simulink library "SimulinkLibrary"  (R2021b)
settings: Solver=VariableStepAuto  StartTime=0.0  StopTime=10.0  RelTol=1e-3
undefined symbols (not defined in the file): Ts, w0
libraries: canmsglib x6, $bdroot x5, sharedtransform x2, simulink x1
(part 1 of 3)
settings Model: Creator=mujim  LastModifiedBy=MujtabaMusa
settings SolverCC: AlgebraicLoopSolver=TrustRegion
settings DebuggingCC: SFMachineParentedDataDiag=warning

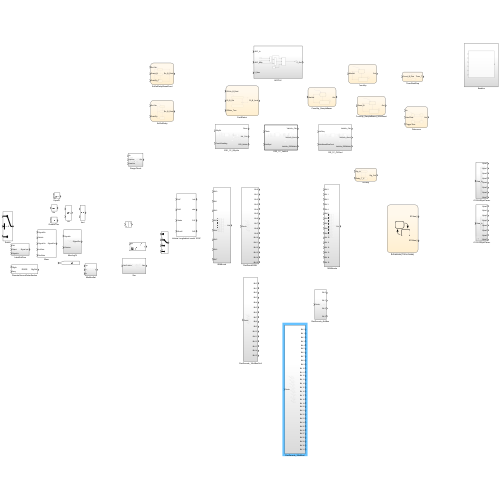
[thumbnail: Simulink's stored preview of the top-level diagram]
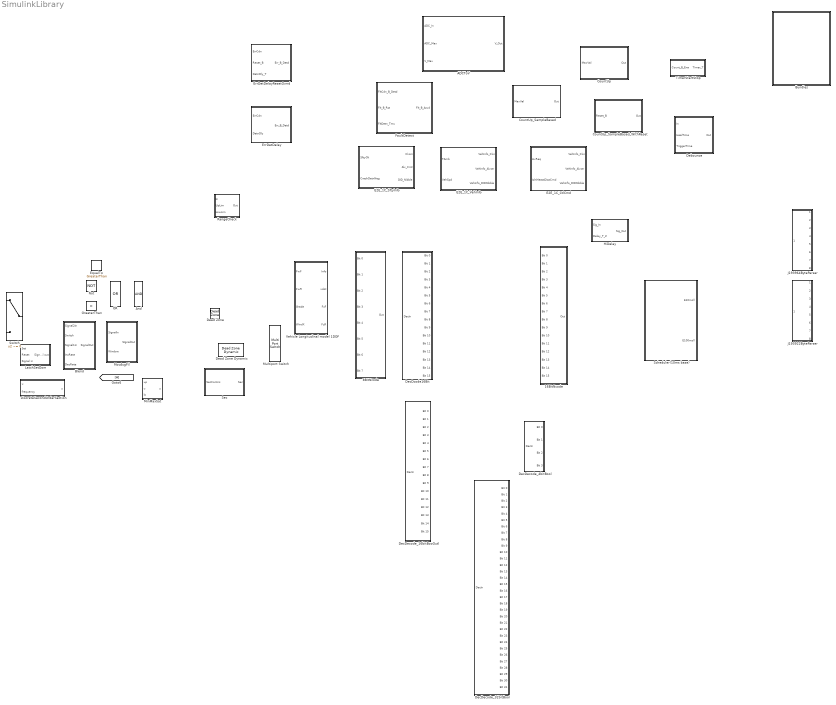
== system SimulinkLibrary ==
  16BitNcode : Subsystem
  8BitNcode : Subsystem
  ADCToV : Subsystem
  And : Logic  AllPortsSameDT=off  OutDataTypeStr=boolean
  Blend : Subsystem  Description=|
      | Blend between 2 signals with a defined rate of rise and fall
      | Switch input:
      | 0 = Signal1
      | 1 = Signal2
      | 
      | Rate is per time step
      mask help:
      | Blend between 2 signals with a defined rate of rise and fall
      | Switch input:
      | 0 = Signal1
      | 1 = Signal2
      |
      | Rate is per time step
      |
      | Use requires a stateflow license
  Bundles : Subsystem
  CountUp : Stateflow chart  TreatAsAtomicUnit=on
  CountUp_SampleBased : Stateflow chart  TreatAsAtomicUnit=on
  CountUp_SampleBased_WithReset : Stateflow chart  TreatAsAtomicUnit=on
  Dead Zone : DeadZone  SaturateOnIntegerOverflow=on
  Dead Zone Dynamic : simulink/Discontinuities/Dead Zone Dynamic
      settings: SourceProductBaseCode=SL
  Debounce : Stateflow chart  TreatAsAtomicUnit=on
  DecDcode16Bit : Subsystem
  DecDecode_16bitBooOutl : Subsystem
  DecDecode_32bitBool : Subsystem
  DecDecode_4bitBool : Subsystem
  DiscreteSecondOrderSection : Subsystem  mask(DiscreteSecondOrderSection){zeta=sin(1*pi/4), Ts=Ts, w0=w0}
      mask prompts: zeta "Damping ratio"; Ts "Sample time Ts"; w0 "Pre-warping frequency w0"
      mask help:
      | Implements the Tustin discretization of the second-order lowpass filter
      |
      |                          w^2
      | F(s) = ---------------------------------------
      |            s^2 + 2 * zeta * w * s + w^2
      |
      | where zeta is the damping ratio and w is the cutoff frequency value fed to the "frequency" port. The discrete transfer function is obtained by Tustin transformation with pre-warping at the frequency w0. The default value w0=0 corresponds to the usual bilinear transformation:
      |
      | s = 2/Ts (z-1)/(z+1).
      mask init:
      | if w0>0
      |    tau = tan(w0*Ts/2)/w0;
      | else
      |    tau = Ts/2;
      | end
      mask Display:
      | text(0.4,0.5,'DSOS');
      | port_label('input', 1, 'SigIn');
      | port_label('output', 1, 'SigOut');
      | port_label('input', 2, 'freq');
  E2E_1C_CtlCmd : Subsystem
  E2E_1C_SftyInfo : Subsystem
  E2E_1C_VehInfo : Subsystem  TreatAsAtomicUnit=on
  EqualTo : $bdroot/GreaterThan  Operator===  OutDataTypeStr=boolean  SampleTime=-1  RndMeth=Zero
  ErrDetDelay : Stateflow chart  TreatAsAtomicUnit=on
  ErrDetDelayResetOvrrd : Stateflow chart  TreatAsAtomicUnit=on
  FaultDetect : Stateflow chart  TreatAsAtomicUnit=on
  GreaterThan : RelationalOperator  Operator=>  OutDataTypeStr=boolean  RndMeth=Zero
  HiDelay : Stateflow chart  TreatAsAtomicUnit=on
  J193922ByteParser : Subsystem  AncestorBlock=SimulinkLibrary/J193964ByteParser
  J193964ByteParser : Subsystem
  LatchSetDom : Subsystem
  MinMaxSat : Subsystem
  MovAvgFil : Subsystem
  Multiport Switch : MultiPortSwitch  Inputs=2  DataPortForDefault=Additional data port  DiagnosticForDefault=None  RndMeth=Zero
  Not : Logic  Operator=NOT  OutDataTypeStr=boolean
  OR : Logic  Operator=OR  AllPortsSameDT=off  OutDataTypeStr=boolean
  RangeCheck : Subsystem
  Scheduler(10ms base) : Stateflow chart  TreatAsAtomicUnit=on
      settings: RTWMemSecFuncInitTerm=Default  RTWMemSecFuncExecute=Default
  Sec : Subsystem
  Switch : Switch  Criteria=u2 ~= 0  OutDataTypeStr=double  RndMeth=Zero
  TimerStartStop : Stateflow chart  TreatAsAtomicUnit=on
  Vehicle Longitudinal model 1DOF : Subsystem  mask(Vehicle Longitudinal model 1DOF){NF=0, NR=0, m=0, a=0, b=0, h=0, Cd=0, Cl=0, Cpm=0, Af=0, x_o=0, xdot_o=0, Pabs=0, T=0, g=0}
      mask prompts: NF "Number of wheels on front axle, NF [-]"; NR "Number of wheels on rear axle, NR [-]"; m "Mass, m [Kg]"; a "Horizontal distance from CG to front axle, a [m]"; b "Horizontal distance from CG to rear axle, b [m]"; h "CG height above axles, h [m]"; Cd "Drag coefficient, Cd [-]"; Cl "Lift coefficient, Cl [-]"; Cpm "Pitch drag moment coeffiecient, Cpm [-]"; Af "Frontal Area, Af [m^2]"; x_o "Initial position, x_o [m]"; xdot_o "Initial velocity, xdot_o [m/s]"; Pabs "Absolute Pressure, Pabs [Pa]"; T "Air Temp, T [K]"; g "Gravitational acceleration, g [m/s^2]"
      mask DialogControl Container3 Prompt: Parameters
      mask DialogControl Container4 Prompt: Vehicle Paramters
      mask DialogControl Container11 Prompt: Environmental Parameters

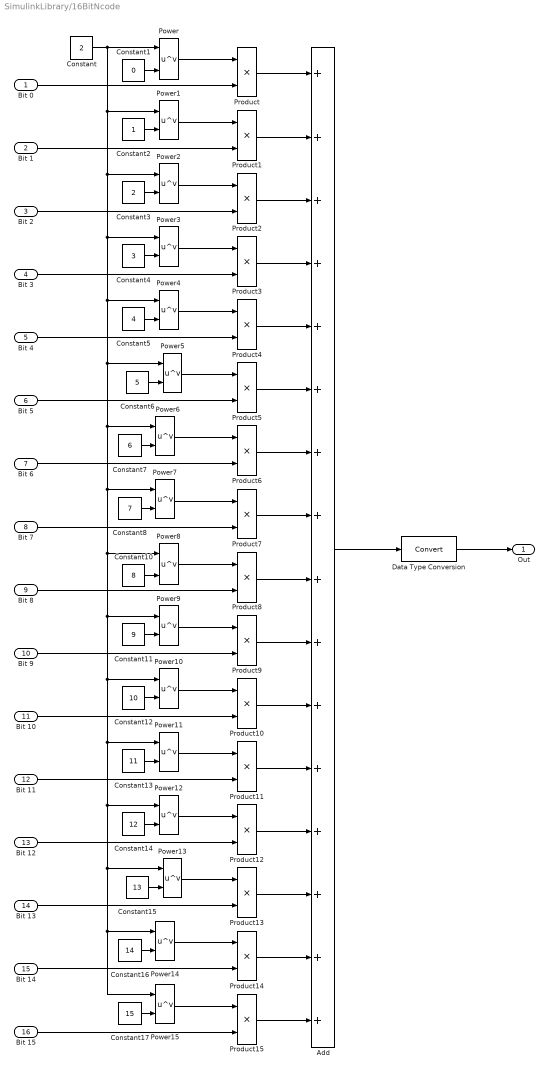
== system SimulinkLibrary/16BitNcode ==
  Bit 0 : Inport  OutDataTypeStr=boolean
  Bit 1 : Inport  Port=2  OutDataTypeStr=boolean
  Bit 2 : Inport  Port=3  OutDataTypeStr=boolean
  Bit 3 : Inport  Port=4  OutDataTypeStr=boolean
  Bit 4 : Inport  Port=5  OutDataTypeStr=boolean
  Bit 5 : Inport  Port=6  OutDataTypeStr=boolean
  Bit 6 : Inport  Port=7  OutDataTypeStr=boolean
  Bit 7 : Inport  Port=8  OutDataTypeStr=boolean
  Bit 8 : Inport  Port=9  OutDataTypeStr=boolean
  Bit 9 : Inport  Port=10  OutDataTypeStr=boolean
  Bit 10 : Inport  Port=11  OutDataTypeStr=boolean
  Bit 11 : Inport  Port=12  OutDataTypeStr=boolean
  Bit 12 : Inport  Port=13  OutDataTypeStr=boolean
  Bit 13 : Inport  Port=14  OutDataTypeStr=boolean
  Bit 14 : Inport  Port=15  OutDataTypeStr=boolean
  Bit 15 : Inport  Port=16  OutDataTypeStr=boolean
  Add : Sum  Inputs=++++++++++++++++
  Constant : Constant  Value=2  OutDataTypeStr=single
  Constant1 : Constant  Value=0  OutDataTypeStr=single
  Constant10 : Constant  Value=8  OutDataTypeStr=single
  Constant11 : Constant  Value=9  OutDataTypeStr=single
  Constant12 : Constant  Value=10  OutDataTypeStr=single
  Constant13 : Constant  Value=11  OutDataTypeStr=single
  Constant14 : Constant  Value=12  OutDataTypeStr=single
  Constant15 : Constant  Value=13  OutDataTypeStr=single
  Constant16 : Constant  Value=14  OutDataTypeStr=single
  Constant17 : Constant  Value=15  OutDataTypeStr=single
  Constant2 : Constant  OutDataTypeStr=single
  Constant3 : Constant  Value=2  OutDataTypeStr=single
  Constant4 : Constant  Value=3  OutDataTypeStr=single
  Constant5 : Constant  Value=4  OutDataTypeStr=single
  Constant6 : Constant  Value=5  OutDataTypeStr=single
  Constant7 : Constant  Value=6  OutDataTypeStr=single
  Constant8 : Constant  Value=7  OutDataTypeStr=single
  Data Type Conversion : DataTypeConversion
  Power{,1..15} (16 alike) : Math  Operator=pow  SaturateOnIntegerOverflow=on
  Product{,1..15} (16 alike) : Product
  Out : Outport
  wires:
  Bit 6/1 -> Product6/2
  Bit 5/1 -> Product5/2
  Product1/1 -> Add/2
  Product/1 -> Add/1
  Bit 1/1 -> Product1/2
  Product7/1 -> Add/8
  Power2/1 -> Product2/1
  Power7/1 -> Product7/1
  Power4/1 -> Product4/1
  Power1/1 -> Product1/1
  Power3/1 -> Product3/1
  Constant4/1 -> Power3/2
  Constant2/1 -> Power1/2
  Constant6/1 -> Power5/2
  Bit 7/1 -> Product7/2
  Constant3/1 -> Power2/2
  Bit 3/1 -> Product3/2
  Bit 4/1 -> Product4/2
  Add/1 -> Data Type Conversion/1
  Power6/1 -> Product6/1
  Constant1/1 -> Power/2
  Bit 2/1 -> Product2/2
  Power5/1 -> Product5/1
  Constant8/1 -> Power7/2
  Bit 0/1 -> Product/2
  Product3/1 -> Add/4
  Product2/1 -> Add/3
  Product4/1 -> Add/5
  Product6/1 -> Add/7
  Constant7/1 -> Power6/2
  Data Type Conversion/1 -> Out/1
  Product5/1 -> Add/6
  Power/1 -> Product/1
  Constant5/1 -> Power4/2
  Product12/1 -> Add/13
  Constant16/1 -> Power14/2
  Product13/1 -> Add/14
  Power8/1 -> Product8/1
  Constant17/1 -> Power15/2
  Product10/1 -> Add/11
  Product11/1 -> Add/12
  Constant14/1 -> Power12/2
  Power13/1 -> Product13/1
  Constant15/1 -> Power13/2
  Constant12/1 -> Power10/2
  Constant/1 -> Power/1, Power1/1, Power2/1, Power3/1, Power8/1, Power9/1, Power10/1, Power11/1, Power15/1, Power14/1, Power13/1, Power12/1, Power7/1, Power6/1, Power5/1, Power4/1
  Product14/1 -> Add/15
  Constant13/1 -> Power11/2
  Constant11/1 -> Power9/2
  Bit 10/1 -> Product10/2
  Power11/1 -> Product11/1
  Constant10/1 -> Power8/2
  Power12/1 -> Product12/1
  Power9/1 -> Product9/1
  Bit 12/1 -> Product12/2
  Power15/1 -> Product15/1
  Bit 15/1 -> Product15/2
  Bit 11/1 -> Product11/2
  Power10/1 -> Product10/1
  Bit 9/1 -> Product9/2
  Product15/1 -> Add/16
  Product9/1 -> Add/10
  Power14/1 -> Product14/1
  Bit 13/1 -> Product13/2
  Bit 14/1 -> Product14/2
  Product8/1 -> Add/9
  Bit 8/1 -> Product8/2

== system SimulinkLibrary/8BitNcode ==
  Bit 0 : Inport  OutDataTypeStr=boolean
  Bit 1 : Inport  Port=2  OutDataTypeStr=boolean
  Bit 2 : Inport  Port=3  OutDataTypeStr=boolean
  Bit 3 : Inport  Port=4  OutDataTypeStr=boolean
  Bit 4 : Inport  Port=5  OutDataTypeStr=boolean
  Bit 5 : Inport  Port=6  OutDataTypeStr=boolean
  Bit 6 : Inport  Port=7  OutDataTypeStr=boolean
  Bit 7 : Inport  Port=8  OutDataTypeStr=boolean
  Add : Sum  Inputs=++++++++
  Constant : Constant  Value=2  OutDataTypeStr=single
  Constant1 : Constant  Value=0  OutDataTypeStr=single
  Constant2 : Constant  OutDataTypeStr=single
  Constant3 : Constant  Value=2  OutDataTypeStr=single
  Constant4 : Constant  Value=3  OutDataTypeStr=single
  Constant5 : Constant  Value=4  OutDataTypeStr=single
  Constant6 : Constant  Value=5  OutDataTypeStr=single
  Constant7 : Constant  Value=6  OutDataTypeStr=single
  Constant8 : Constant  Value=7  OutDataTypeStr=single
  Data Type Conversion : DataTypeConversion
  Power{,1..7} (8 alike) : Math  Operator=pow  SaturateOnIntegerOverflow=on
  Product{,1..7} (8 alike) : Product
  Out : Outport
  wires:
  Bit 0/1 -> Product/2
  Constant/1 -> Power/1, Power1/1, Power2/1, Power3/1, Power7/1, Power6/1, Power5/1, Power4/1
  Power/1 -> Product/1
  Add/1 -> Data Type Conversion/1
  Constant1/1 -> Power/2
  Constant2/1 -> Power1/2
  Constant3/1 -> Power2/2
  Constant4/1 -> Power3/2
  Constant5/1 -> Power4/2
  Constant6/1 -> Power5/2
  Constant7/1 -> Power6/2
  Constant8/1 -> Power7/2
  Product/1 -> Add/1
  Product1/1 -> Add/2
  Product2/1 -> Add/3
  Product3/1 -> Add/4
  Product4/1 -> Add/5
  Product5/1 -> Add/6
  Product6/1 -> Add/7
  Product7/1 -> Add/8
  Power1/1 -> Product1/1
  Power2/1 -> Product2/1
  Power3/1 -> Product3/1
  Power4/1 -> Product4/1
  Power5/1 -> Product5/1
  Power6/1 -> Product6/1
  Power7/1 -> Product7/1
  Bit 1/1 -> Product1/2
  Bit 2/1 -> Product2/2
  Bit 3/1 -> Product3/2
  Bit 4/1 -> Product4/2
  Bit 5/1 -> Product5/2
  Bit 6/1 -> Product6/2
  Bit 7/1 -> Product7/2
  Data Type Conversion/1 -> Out/1

== system SimulinkLibrary/ADCToV ==
  ADC_In : Inport
  ADC_Max : Inport  Port=2
  V_Max : Inport  Port=3
  Constant : Constant  Value=0
  Divide : Product  Inputs=*/
  MinMaxSat : $bdroot/MinMaxSat  SystemSampleTime=-1  VariantActivationTime=update diagram  Latency=0  AutoFrameSizeCalculation=off
  Product : Product
  V_Out : Outport
  wires:
  Constant/1 -> MinMaxSat/3
  MinMaxSat/1 -> V_Out/1  "V_Out"
  Product/1 -> MinMaxSat/2
  V_Max/1 -> Product/2, MinMaxSat/1  "V_Max"
  Divide/1 -> Product/1
  ADC_In/1 -> Divide/1  "ADC_In"
  ADC_Max/1 -> Divide/2  "ADC_Max"

== system SimulinkLibrary/Blend ==
  note: Blend between 2 signals with a defined rate of rise and fall
      | Switch input:
      | 0 = Signal1
      | 1 = Signal2
      |
      | Rate is per time step
  Signal2In : Inport
  Switch : Inport  Port=2
  Signal1In : Inport  Port=3
  IncRate : Inport  Port=4
  DecRate : Inport  Port=5
  Chart : Stateflow chart  TreatAsAtomicUnit=on
  SignalOut : Outport
  wires:
  Signal2In/1 -> Chart/3(SigIn2)
  Signal1In/1 -> Chart/2(SigIn1)
  DecRate/1 -> Chart/5(DecRate)
  Switch/1 -> Chart/1(Swt)
  IncRate/1 -> Chart/4(IncRate)
  Chart/1(SigOut) -> SignalOut/1

== system SimulinkLibrary/Bundles ==
  HwSelProc : Subsystem

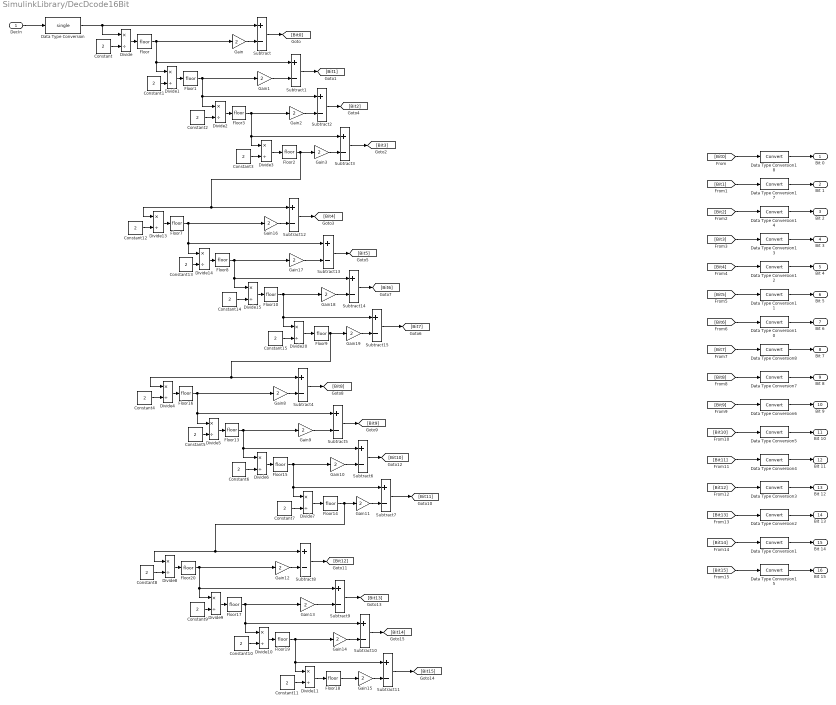
== system SimulinkLibrary/DecDcode16Bit ==
  DecIn : Inport
  Constant{,1..15} (16 alike) : Constant  Value=2  OutDataTypeStr=single
  Data Type Conversion : DataTypeConversion  OutDataTypeStr=single
  Data Type Conversion{1..8,10..15,17..18} (16 alike) : DataTypeConversion
  Divide{,1..11,13..15,20} (16 alike) : Product  Inputs=*/  OutDataTypeStr=Inherit: Inherit via back propagation
  Floor{,1..3,7..10,13..20} (16 alike) : Rounding
  Gain{,1..3,8..19} (16 alike) : Gain  Gain=2
  Subtract{,1..15} (16 alike) : Sum  Inputs=+-
  Bit 0 : Outport
  Bit 1 : Outport  Port=2
  Bit 2 : Outport  Port=3
  Bit 3 : Outport  Port=4
  Bit 4 : Outport  Port=5
  Bit 5 : Outport  Port=6
  Bit 6 : Outport  Port=7
  Bit 7 : Outport  Port=8
  Bit 8 : Outport  Port=9
  Bit 9 : Outport  Port=10
  Bit 10 : Outport  Port=11
  Bit 11 : Outport  Port=12
  Bit 12 : Outport  Port=13
  Bit 13 : Outport  Port=14
  Bit 14 : Outport  Port=15
  Bit 15 : Outport  Port=16
  wires:
  Constant/1 -> Divide/2
  Divide/1 -> Floor/1
  Divide1/1 -> Floor1/1
  Constant1/1 -> Divide1/2
  Subtract/1 -> [Bit0]
  Constant2/1 -> Divide2/2
  Divide2/1 -> Floor3/1
  [Bit0] -> Data Type Conversion18/1
  Subtract1/1 -> [Bit1]
  [Bit1] -> Data Type Conversion17/1
  Subtract3/1 -> [Bit3]
  Constant3/1 -> Divide3/2
  Subtract2/1 -> [Bit2]
  [Bit2] -> Data Type Conversion14/1
  [Bit3] -> Data Type Conversion13/1
  [Bit4] -> Data Type Conversion12/1
  [Bit5] -> Data Type Conversion11/1
  [Bit6] -> Data Type Conversion10/1
  [Bit7] -> Data Type Conversion8/1
  [Bit15] -> Data Type Conversion15/1
  [Bit14] -> Data Type Conversion1/1
  [Bit13] -> Data Type Conversion2/1
  [Bit12] -> Data Type Conversion3/1
  [Bit11] -> Data Type Conversion4/1
  [Bit10] -> Data Type Conversion5/1
  [Bit9] -> Data Type Conversion6/1
  [Bit8] -> Data Type Conversion7/1
  Gain/1 -> Subtract/2
  Gain1/1 -> Subtract1/2
  Gain2/1 -> Subtract2/2
  Gain3/1 -> Subtract3/2
  Divide3/1 -> Floor2/1
  Data Type Conversion18/1 -> Bit 0/1
  Data Type Conversion17/1 -> Bit 1/1
  Data Type Conversion14/1 -> Bit 2/1
  Data Type Conversion13/1 -> Bit 3/1
  Data Type Conversion12/1 -> Bit 4/1
  Data Type Conversion11/1 -> Bit 5/1
  Data Type Conversion10/1 -> Bit 6/1
  Data Type Conversion8/1 -> Bit 7/1
  Data Type Conversion7/1 -> Bit 8/1
  Data Type Conversion6/1 -> Bit 9/1
  Data Type Conversion5/1 -> Bit 10/1
  Data Type Conversion4/1 -> Bit 11/1
  Data Type Conversion3/1 -> Bit 12/1
  Data Type Conversion2/1 -> Bit 13/1
  Data Type Conversion1/1 -> Bit 14/1
  Data Type Conversion15/1 -> Bit 15/1
  DecIn/1 -> Data Type Conversion/1
  Floor/1 -> Gain/1, Divide1/1, Subtract1/1
  Floor1/1 -> Gain1/1, Divide2/1, Subtract2/1
  Floor3/1 -> Gain2/1, Divide3/1, Subtract3/1
  Floor10/1 -> Subtract15/1, Divide20/1, Gain18/1
  Floor8/1 -> Subtract14/1, Divide15/1, Gain17/1
  Floor7/1 -> Subtract13/1, Divide14/1, Gain16/1
  Floor2/1 -> Divide13/1, Subtract12/1, Gain3/1
  Divide20/1 -> Floor9/1
  Gain19/1 -> Subtract15/2
  Gain18/1 -> Subtract14/2
  Gain17/1 -> Subtract13/2
  Gain16/1 -> Subtract12/2
  Subtract14/1 -> [Bit6]
  Constant15/1 -> Divide20/2
  Subtract15/1 -> [Bit7]
  Subtract13/1 -> [Bit5]
  Divide15/1 -> Floor10/1
  Constant14/1 -> Divide15/2
  Subtract12/1 -> [Bit4]
  Constant13/1 -> Divide14/2
  Divide14/1 -> Floor8/1
  Divide13/1 -> Floor7/1
  Constant12/1 -> Divide13/2
  Floor15/1 -> Subtract7/1, Divide7/1, Gain10/1
  Floor13/1 -> Subtract6/1, Divide6/1, Gain9/1
  Floor16/1 -> Subtract5/1, Divide5/1, Gain8/1
  Floor9/1 -> Gain19/1, Divide4/1, Subtract4/1
  Divide7/1 -> Floor14/1
  Gain11/1 -> Subtract7/2
  Gain10/1 -> Subtract6/2
  Gain9/1 -> Subtract5/2
  Gain8/1 -> Subtract4/2
  Subtract6/1 -> [Bit10]
  Constant7/1 -> Divide7/2
  Subtract7/1 -> [Bit11]
  Subtract5/1 -> [Bit9]
  Divide6/1 -> Floor15/1
  Constant6/1 -> Divide6/2
  Subtract4/1 -> [Bit8]
  Constant5/1 -> Divide5/2
  Divide5/1 -> Floor13/1
  Divide4/1 -> Floor16/1
  Constant4/1 -> Divide4/2
  Floor18/1 -> Gain15/1
  Floor19/1 -> Subtract11/1, Divide11/1, Gain14/1
  Floor17/1 -> Subtract10/1, Divide10/1, Gain13/1
  Floor20/1 -> Subtract9/1, Divide9/1, Gain12/1
  Floor14/1 -> Subtract8/1, Divide8/1, Gain11/1
  Divide11/1 -> Floor18/1
  Gain15/1 -> Subtract11/2
  Gain14/1 -> Subtract10/2
  Gain13/1 -> Subtract9/2
  Gain12/1 -> Subtract8/2
  Subtract10/1 -> [Bit14]
  Constant11/1 -> Divide11/2
  Subtract11/1 -> [Bit15]
  Subtract9/1 -> [Bit13]
  Divide10/1 -> Floor19/1
  Constant10/1 -> Divide10/2
  Subtract8/1 -> [Bit12]
  Constant9/1 -> Divide9/2
  Divide9/1 -> Floor17/1
  Divide8/1 -> Floor20/1
  Constant8/1 -> Divide8/2
  Data Type Conversion/1 -> Divide/1, Subtract/1

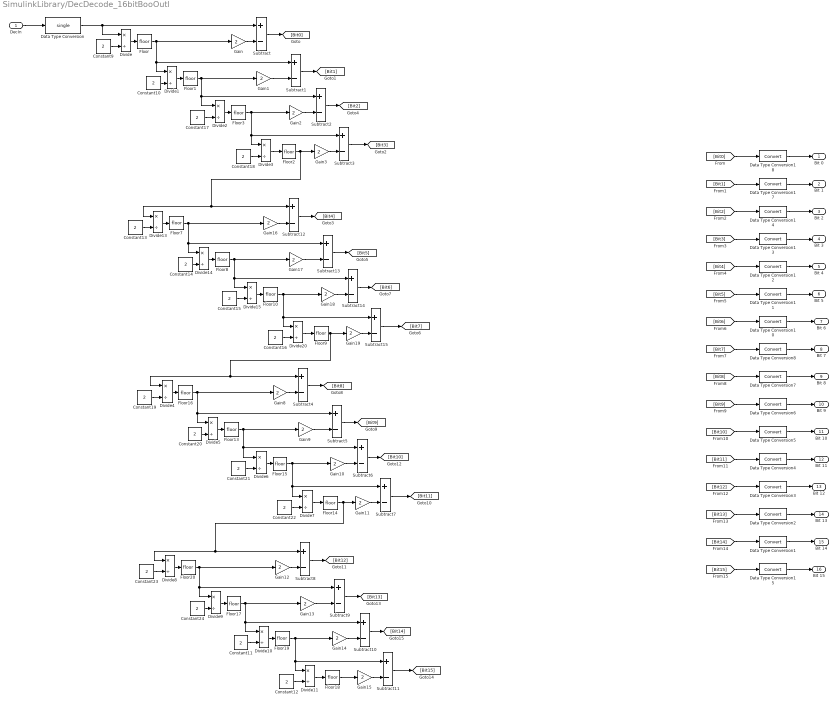
== system SimulinkLibrary/DecDecode_16bitBooOutl ==
  DecIn : Inport
  Constant{9..24} (16 alike) : Constant  Value=2  OutDataTypeStr=single
  Data Type Conversion : DataTypeConversion  OutDataTypeStr=single
  Data Type Conversion{1..8,10..15,17..18} (16 alike) : DataTypeConversion
  Divide{,1..11,13..15,20} (16 alike) : Product  Inputs=*/  OutDataTypeStr=Inherit: Inherit via back propagation
  Floor{,1..3,7..10,13..20} (16 alike) : Rounding
  Gain{,1..3,8..19} (16 alike) : Gain  Gain=2
  Subtract{,1..15} (16 alike) : Sum  Inputs=+-
  Bit 0 : Outport  OutDataTypeStr=boolean
  Bit 1 : Outport  Port=2  OutDataTypeStr=boolean
  Bit 2 : Outport  Port=3  OutDataTypeStr=boolean
  Bit 3 : Outport  Port=4  OutDataTypeStr=boolean
  Bit 4 : Outport  Port=5  OutDataTypeStr=boolean
  Bit 5 : Outport  Port=6  OutDataTypeStr=boolean
  Bit 6 : Outport  Port=7  OutDataTypeStr=boolean
  Bit 7 : Outport  Port=8  OutDataTypeStr=boolean
  Bit 8 : Outport  Port=9  OutDataTypeStr=boolean
  Bit 9 : Outport  Port=10  OutDataTypeStr=boolean
  Bit 10 : Outport  Port=11  OutDataTypeStr=boolean
  Bit 11 : Outport  Port=12  OutDataTypeStr=boolean
  Bit 12 : Outport  Port=13  OutDataTypeStr=boolean
  Bit 13 : Outport  Port=14  OutDataTypeStr=boolean
  Bit 14 : Outport  Port=15  OutDataTypeStr=boolean
  Bit 15 : Outport  Port=16  OutDataTypeStr=boolean
  wires:
  Subtract15/1 -> [Bit7]
  Gain19/1 -> Subtract15/2
  Data Type Conversion17/1 -> Bit 1/1
  Floor8/1 -> Gain17/1, Divide15/1, Subtract14/1
  Gain/1 -> Subtract/2
  Gain17/1 -> Subtract13/2
  Data Type Conversion12/1 -> Bit 4/1
  Subtract9/1 -> [Bit13]
  Divide9/1 -> Floor17/1
  Subtract1/1 -> [Bit1]
  [Bit11] -> Data Type Conversion4/1
  [Bit5] -> Data Type Conversion11/1
  [Bit9] -> Data Type Conversion6/1
  Gain1/1 -> Subtract1/2
  Subtract2/1 -> [Bit2]
  [Bit14] -> Data Type Conversion1/1
  [Bit0] -> Data Type Conversion18/1
  Data Type Conversion14/1 -> Bit 2/1
  Subtract8/1 -> [Bit12]
  Subtract7/1 -> [Bit11]
  [Bit2] -> Data Type Conversion14/1
  [Bit15] -> Data Type Conversion15/1
  Constant10/1 -> Divide1/2
  Subtract/1 -> [Bit0]
  Constant18/1 -> Divide3/2
  Constant16/1 -> Divide20/2
  [Bit1] -> Data Type Conversion17/1
  [Bit10] -> Data Type Conversion5/1
  Divide/1 -> Floor/1
  [Bit3] -> Data Type Conversion13/1
  Constant17/1 -> Divide2/2
  Floor2/1 -> Gain3/1, Subtract12/1, Divide13/1
  Data Type Conversion3/1 -> Bit 12/1
  Data Type Conversion15/1 -> Bit 15/1
  Subtract6/1 -> [Bit10]
  Constant14/1 -> Divide14/2
  Constant15/1 -> Divide15/2
  Gain13/1 -> Subtract9/2
  DecIn/1 -> Data Type Conversion/1
  Subtract5/1 -> [Bit9]
  Floor1/1 -> Subtract2/1, Divide2/1, Gain1/1
  Divide10/1 -> Floor19/1
  Divide13/1 -> Floor7/1
  Data Type Conversion2/1 -> Bit 13/1
  Gain15/1 -> Subtract11/2
  Floor13/1 -> Gain9/1, Divide6/1, Subtract6/1
  Subtract11/1 -> [Bit15]
  Constant19/1 -> Divide4/2
  Constant12/1 -> Divide11/2
  Divide5/1 -> Floor13/1
  Data Type Conversion8/1 -> Bit 7/1
  Floor18/1 -> Gain15/1
  Divide20/1 -> Floor9/1
  Constant20/1 -> Divide5/2
  Floor7/1 -> Gain16/1, Divide14/1, Subtract13/1
  Gain18/1 -> Subtract14/2
  Data Type Conversion1/1 -> Bit 14/1
  Data Type Conversion13/1 -> Bit 3/1
  Divide11/1 -> Floor18/1
  Divide7/1 -> Floor14/1
  Data Type Conversion5/1 -> Bit 10/1
  Data Type Conversion4/1 -> Bit 11/1
  Subtract13/1 -> [Bit5]
  Data Type Conversion7/1 -> Bit 8/1
  Gain3/1 -> Subtract3/2
  Constant22/1 -> Divide7/2
  Data Type Conversion11/1 -> Bit 5/1
  [Bit7] -> Data Type Conversion8/1
  Divide1/1 -> Floor1/1
  Data Type Conversion18/1 -> Bit 0/1
  Divide3/1 -> Floor2/1
  Data Type Conversion10/1 -> Bit 6/1
  Floor/1 -> Subtract1/1, Divide1/1, Gain/1
  Constant9/1 -> Divide/2
  [Bit6] -> Data Type Conversion10/1
  [Bit12] -> Data Type Conversion3/1
  Gain2/1 -> Subtract2/2
  Floor15/1 -> Gain10/1, Divide7/1, Subtract7/1
  Floor9/1 -> Subtract4/1, Divide4/1, Gain19/1
  Gain8/1 -> Subtract4/2
  Gain9/1 -> Subtract5/2
  Gain10/1 -> Subtract6/2
  Floor16/1 -> Gain8/1, Divide5/1, Subtract5/1
  Gain16/1 -> Subtract12/2
  Divide15/1 -> Floor10/1
  Floor10/1 -> Gain18/1, Divide20/1, Subtract15/1
  Floor14/1 -> Gain11/1, Divide8/1, Subtract8/1
  Subtract10/1 -> [Bit14]
  Divide14/1 -> Floor8/1
  Floor20/1 -> Gain12/1, Divide9/1, Subtract9/1
  Floor3/1 -> Subtract3/1, Divide3/1, Gain2/1
  Constant24/1 -> Divide9/2
  Divide2/1 -> Floor3/1
  Divide6/1 -> Floor15/1
  Floor17/1 -> Gain13/1, Divide10/1, Subtract10/1
  Constant13/1 -> Divide13/2
  [Bit8] -> Data Type Conversion7/1
  Gain14/1 -> Subtract10/2
  [Bit4] -> Data Type Conversion12/1
  Constant11/1 -> Divide10/2
  Subtract4/1 -> [Bit8]
  Floor19/1 -> Gain14/1, Divide11/1, Subtract11/1
  Constant21/1 -> Divide6/2
  Subtract12/1 -> [Bit4]
  Subtract3/1 -> [Bit3]
  Divide4/1 -> Floor16/1
  Data Type Conversion/1 -> Subtract/1, Divide/1
  [Bit13] -> Data Type Conversion2/1
  Divide8/1 -> Floor20/1
  Gain12/1 -> Subtract8/2
  Data Type Conversion6/1 -> Bit 9/1
  Gain11/1 -> Subtract7/2
  Subtract14/1 -> [Bit6]
  Constant23/1 -> Divide8/2

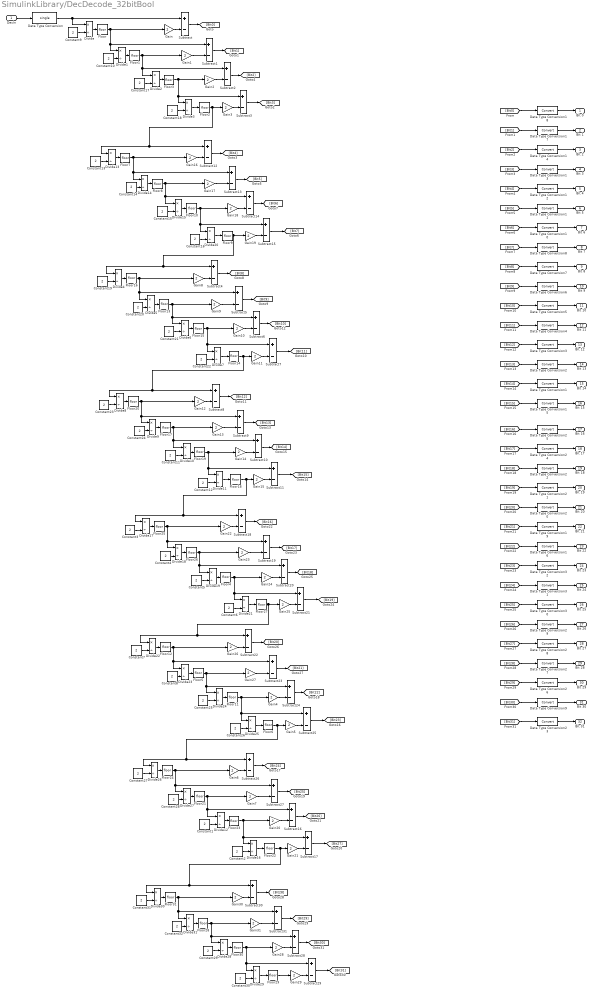
== system SimulinkLibrary/DecDecode_32bitBool ==
  DecIn : Inport
  Constant{1..32} (32 alike) : Constant  Value=2  OutDataTypeStr=single
  Data Type Conversion : DataTypeConversion  OutDataTypeStr=single
  Data Type Conversion{1..32} (32 alike) : DataTypeConversion
  Divide{,1..31} (32 alike) : Product  Inputs=*/  OutDataTypeStr=Inherit: Inherit via back propagation
  Floor{,1..31} (32 alike) : Rounding
  Gain{,1..31} (32 alike) : Gain  Gain=2
  Subtract{,1..31} (32 alike) : Sum  Inputs=+-
  Bit 0 : Outport  OutDataTypeStr=boolean
  Bit 1 : Outport  Port=2  OutDataTypeStr=boolean
  Bit 2 : Outport  Port=3  OutDataTypeStr=boolean
  Bit 3 : Outport  Port=4  OutDataTypeStr=boolean
  Bit 4 : Outport  Port=5  OutDataTypeStr=boolean
  Bit 5 : Outport  Port=6  OutDataTypeStr=boolean
  Bit 6 : Outport  Port=7  OutDataTypeStr=boolean
  Bit 7 : Outport  Port=8  OutDataTypeStr=boolean
  Bit 8 : Outport  Port=9  OutDataTypeStr=boolean
  Bit 9 : Outport  Port=10  OutDataTypeStr=boolean
  Bit 10 : Outport  Port=11  OutDataTypeStr=boolean
  Bit 11 : Outport  Port=12  OutDataTypeStr=boolean
  Bit 12 : Outport  Port=13  OutDataTypeStr=boolean
  Bit 13 : Outport  Port=14  OutDataTypeStr=boolean
  Bit 14 : Outport  Port=15  OutDataTypeStr=boolean
  Bit 15 : Outport  Port=16  OutDataTypeStr=boolean
  Bit 16 : Outport  Port=17  OutDataTypeStr=boolean
  Bit 17 : Outport  Port=18  OutDataTypeStr=boolean
  Bit 18 : Outport  Port=19  OutDataTypeStr=boolean
  Bit 19 : Outport  Port=20  OutDataTypeStr=boolean
  Bit 20 : Outport  Port=21  OutDataTypeStr=boolean
  Bit 21 : Outport  Port=22  OutDataTypeStr=boolean
  Bit 22 : Outport  Port=23  OutDataTypeStr=boolean
  Bit 23 : Outport  Port=24  OutDataTypeStr=boolean
  Bit 24 : Outport  Port=25  OutDataTypeStr=boolean
  Bit 25 : Outport  Port=26  OutDataTypeStr=boolean
  Bit 26 : Outport  Port=27  OutDataTypeStr=boolean
  Bit 27 : Outport  Port=28  OutDataTypeStr=boolean
  Bit 28 : Outport  Port=29  OutDataTypeStr=boolean
  Bit 29 : Outport  Port=30  OutDataTypeStr=boolean
  Bit 30 : Outport  Port=31  OutDataTypeStr=boolean
  Bit 31 : Outport  Port=32  OutDataTypeStr=boolean
  wires:
  Subtract4/1 -> [Bit8]
  Data Type Conversion6/1 -> Bit 9/1
  Constant23/1 -> Divide8/2
  Constant17/1 -> Divide2/2
  Constant19/1 -> Divide4/2
  Data Type Conversion13/1 -> Bit 3/1
  Floor7/1 -> Gain16/1, Divide14/1, Subtract13/1
  Divide11/1 -> Floor18/1
  Gain18/1 -> Subtract14/2
  Data Type Conversion4/1 -> Bit 11/1
  [Bit7] -> Data Type Conversion8/1
  Constant22/1 -> Divide7/2
  Constant20/1 -> Divide5/2
  Subtract11/1 -> [Bit15]
  Constant12/1 -> Divide11/2
  Data Type Conversion2/1 -> Bit 13/1
  Divide5/1 -> Floor13/1
  Gain15/1 -> Subtract11/2
  Divide10/1 -> Floor19/1
  Subtract5/1 -> [Bit9]
  Data Type Conversion15/1 -> Bit 15/1
  Gain13/1 -> Subtract9/2
  Gain17/1 -> Subtract13/2
  DecIn/1 -> Data Type Conversion/1
  [Bit10] -> Data Type Conversion5/1
  [Bit2] -> Data Type Conversion14/1
  Constant18/1 -> Divide3/2
  Subtract/1 -> [Bit0]
  Constant10/1 -> Divide1/2
  Divide/1 -> Floor/1
  Floor8/1 -> Gain17/1, Divide15/1, Subtract14/1
  [Bit1] -> Data Type Conversion17/1
  Data Type Conversion3/1 -> Bit 12/1
  [Bit11] -> Data Type Conversion4/1
  Subtract1/1 -> [Bit1]
  Gain1/1 -> Subtract1/2
  Subtract7/1 -> [Bit11]
  [Bit14] -> Data Type Conversion1/1
  Data Type Conversion12/1 -> Bit 4/1
  Data Type Conversion14/1 -> Bit 2/1
  Subtract15/1 -> [Bit7]
  Gain/1 -> Subtract/2
  Data Type Conversion17/1 -> Bit 1/1
  Constant24/1 -> Divide9/2
  Data Type Conversion1/1 -> Bit 14/1
  Floor13/1 -> Gain9/1, Divide6/1, Subtract6/1
  Floor20/1 -> Gain12/1, Divide9/1, Subtract9/1
  Floor14/1 -> Gain11/1, Divide8/1, Subtract8/1
  Subtract10/1 -> [Bit14]
  Floor10/1 -> Gain18/1, Divide20/1, Subtract15/1
  Data Type Conversion18/1 -> Bit 0/1
  Gain2/1 -> Subtract2/2
  Gain19/1 -> Subtract15/2
  Data Type Conversion7/1 -> Bit 8/1
  Data Type Conversion8/1 -> Bit 7/1
  Gain10/1 -> Subtract6/2
  Gain16/1 -> Subtract12/2
  [Bit15] -> Data Type Conversion15/1
  Subtract6/1 -> [Bit10]
  Subtract9/1 -> [Bit13]
  Gain3/1 -> Subtract3/2
  Divide15/1 -> Floor10/1
  Divide3/1 -> Floor2/1
  Floor/1 -> Subtract1/1, Divide1/1, Gain/1
  [Bit6] -> Data Type Conversion10/1
  Subtract14/1 -> [Bit6]
  Constant9/1 -> Divide/2
  Constant16/1 -> Divide20/2
  Subtract2/1 -> [Bit2]
  Data Type Conversion11/1 -> Bit 5/1
  Gain11/1 -> Subtract7/2
  Constant11/1 -> Divide10/2
  Floor9/1 -> Subtract4/1, Divide4/1, Gain19/1
  Data Type Conversion5/1 -> Bit 10/1
  Gain8/1 -> Subtract4/2
  Data Type Conversion/1 -> Subtract/1, Divide/1
  Floor15/1 -> Gain10/1, Divide7/1, Subtract7/1
  Subtract3/1 -> [Bit3]
  [Bit8] -> Data Type Conversion7/1
  Floor2/1 -> Gain3/1, Subtract12/1, Divide13/1
  Divide4/1 -> Floor16/1
  [Bit5] -> Data Type Conversion11/1
  Floor3/1 -> Subtract3/1, Divide3/1, Gain2/1
  Divide9/1 -> Floor17/1
  Data Type Conversion10/1 -> Bit 6/1
  Constant15/1 -> Divide15/2
  [Bit4] -> Data Type Conversion12/1
  Divide7/1 -> Floor14/1
  Subtract13/1 -> [Bit5]
  Constant21/1 -> Divide6/2
  Floor16/1 -> Gain8/1, Divide5/1, Subtract5/1
  Subtract8/1 -> [Bit12]
  Subtract12/1 -> [Bit4]
  Divide1/1 -> Floor1/1
  Floor1/1 -> Subtract2/1, Divide2/1, Gain1/1
  Divide2/1 -> Floor3/1
  Gain12/1 -> Subtract8/2
  Constant13/1 -> Divide13/2
  Constant14/1 -> Divide14/2
  [Bit9] -> Data Type Conversion6/1
  [Bit12] -> Data Type Conversion3/1
  [Bit3] -> Data Type Conversion13/1
  Gain14/1 -> Subtract10/2
  [Bit13] -> Data Type Conversion2/1
  Divide14/1 -> Floor8/1
  Gain9/1 -> Subtract5/2
  [Bit0] -> Data Type Conversion18/1
  Divide20/1 -> Floor9/1
  Divide6/1 -> Floor15/1
  Divide13/1 -> Floor7/1
  Floor17/1 -> Gain13/1, Divide10/1, Subtract10/1
  Floor19/1 -> Gain14/1, Divide11/1, Subtract11/1
  Divide8/1 -> Floor20/1
  Subtract25/1 -> [Bit23]
  Gain25/1 -> Subtract21/2
  Subtract16/1 -> [Bit26]
  Floor6/1 -> Gain5/1, Divide26/1, Subtract26/1
  Floor24/1 -> Gain6/1, Divide27/1, Subtract27/1
  Floor5/1 -> Gain27/1, Divide24/1, Subtract24/1
  Constant28/1 -> Divide27/2
  Subtract21/1 -> [Bit19]
  Gain26/1 -> Subtract22/2
  Floor27/1 -> Subtract22/1, Divide22/1, Gain25/1
  Constant1/1 -> Divide12/2
  Gain5/1 -> Subtract25/2
  Constant6/1 -> Divide21/2
  Subtract20/1 -> [Bit18]
  Divide19/1 -> Floor4/1
  Subtract27/1 -> [Bit25]
  Subtract24/1 -> [Bit22]
  Gain22/1 -> Subtract18/2
  Gain4/1 -> Subtract24/2
  Divide25/1 -> Floor6/1
  Constant5/1 -> Divide19/2
  Divide27/1 -> Floor21/1
  Constant25/1 -> Divide24/2
  Floor11/1 -> Gain4/1, Divide25/1, Subtract25/1
  Subtract18/1 -> [Bit16]
  Floor12/1 -> Gain26/1, Divide23/1, Subtract23/1
  Floor26/1 -> Gain23/1, Divide19/1, Subtract20/1
  Gain7/1 -> Subtract27/2
  Divide23/1 -> Floor5/1
  Gain21/1 -> Subtract17/2
  Subtract26/1 -> [Bit24]
  Divide12/1 -> Floor23/1
  Floor4/1 -> Gain24/1, Divide21/1, Subtract21/1
  Gain23/1 -> Subtract19/2
  Divide16/1 -> Floor22/1
  Gain24/1 -> Subtract20/2
  Floor25/1 -> Gain22/1, Divide18/1, Subtract19/1
  Constant7/1 -> Divide22/2
  Subtract22/1 -> [Bit20]
  Constant26/1 -> Divide25/2
  Subtract17/1 -> [Bit27]
  Gain27/1 -> Subtract23/2
  Gain20/1 -> Subtract16/2
  Divide18/1 -> Floor26/1
  Constant4/1 -> Divide18/2
  Constant3/1 -> Divide17/2
  Floor23/1 -> Gain20/1, Divide16/1, Subtract17/1
  Constant8/1 -> Divide23/2
  Subtract19/1 -> [Bit17]
  Divide26/1 -> Floor24/1
  Divide22/1 -> Floor12/1
  Divide17/1 -> Floor25/1
  Divide21/1 -> Floor27/1
  Constant27/1 -> Divide26/2
  Floor21/1 -> Gain7/1, Divide12/1, Subtract16/1
  Gain6/1 -> Subtract26/2
  Subtract23/1 -> [Bit21]
  Divide24/1 -> Floor11/1
  Constant2/1 -> Divide16/2
  Floor18/1 -> Subtract18/1, Divide17/1, Gain15/1
  Constant32/1 -> Divide31/2
  Floor31/1 -> Gain30/1, Divide31/1, Subtract31/1
  Floor22/1 -> Divide30/1, Subtract30/1, Gain21/1
  Subtract28/1 -> [Bit30]
  Floor30/1 -> Gain28/1, Divide29/1, Subtract29/1
  Floor29/1 -> Gain29/1
  Divide29/1 -> Floor29/1
  Gain31/1 -> Subtract31/2
  Subtract30/1 -> [Bit28]
  Gain29/1 -> Subtract29/2
  Divide31/1 -> Floor28/1
  Subtract29/1 -> [Bit31]
  Subtract31/1 -> [Bit29]
  Constant29/1 -> Divide28/2
  Constant30/1 -> Divide29/2
  Floor28/1 -> Gain31/1, Divide28/1, Subtract28/1
  Gain30/1 -> Subtract30/2
  Divide28/1 -> Floor30/1
  Constant31/1 -> Divide30/2
  Gain28/1 -> Subtract28/2
  Divide30/1 -> Floor31/1
  Data Type Conversion25/1 -> Bit 16/1
  Data Type Conversion9/1 -> Bit 30/1
  Data Type Conversion24/1 -> Bit 17/1
  Data Type Conversion20/1 -> Bit 20/1
  Data Type Conversion22/1 -> Bit 18/1
  Data Type Conversion29/1 -> Bit 26/1
  Data Type Conversion31/1 -> Bit 24/1
  Data Type Conversion32/1 -> Bit 23/1
  Data Type Conversion16/1 -> Bit 22/1
  Data Type Conversion27/1 -> Bit 28/1
  Data Type Conversion23/1 -> Bit 31/1
  Data Type Conversion21/1 -> Bit 19/1
  Data Type Conversion19/1 -> Bit 21/1
  Data Type Conversion28/1 -> Bit 27/1
  Data Type Conversion30/1 -> Bit 25/1
  Data Type Conversion26/1 -> Bit 29/1
  [Bit16] -> Data Type Conversion25/1
  [Bit17] -> Data Type Conversion24/1
  [Bit18] -> Data Type Conversion22/1
  [Bit19] -> Data Type Conversion21/1
  [Bit20] -> Data Type Conversion20/1
  [Bit21] -> Data Type Conversion19/1
  [Bit22] -> Data Type Conversion16/1
  [Bit23] -> Data Type Conversion32/1
  [Bit24] -> Data Type Conversion31/1
  [Bit25] -> Data Type Conversion30/1
  [Bit26] -> Data Type Conversion29/1
  [Bit27] -> Data Type Conversion28/1
  [Bit28] -> Data Type Conversion27/1
  [Bit29] -> Data Type Conversion26/1
  [Bit30] -> Data Type Conversion9/1
  [Bit31] -> Data Type Conversion23/1

== system SimulinkLibrary/DecDecode_4bitBool ==
  DecIn : Inport
  Constant{9..10,17..18} (4 alike) : Constant  Value=2  OutDataTypeStr=single
  Data Type Conversion : DataTypeConversion  OutDataTypeStr=single
  Data Type Conversion{13..14,17..18} (4 alike) : DataTypeConversion
  Divide{,1..3} (4 alike) : Product  Inputs=*/  OutDataTypeStr=Inherit: Inherit via back propagation
  Floor{,1..3} (4 alike) : Rounding
  Gain{,1..3} (4 alike) : Gain  Gain=2
  Subtract{,1..3} (4 alike) : Sum  Inputs=+-
  Bit 0 : Outport  OutDataTypeStr=boolean
  Bit 1 : Outport  Port=2  OutDataTypeStr=boolean
  Bit 2 : Outport  Port=3  OutDataTypeStr=boolean
  Bit 3 : Outport  Port=4  OutDataTypeStr=boolean
  wires:
  Data Type Conversion/1 -> Divide/1, Subtract/1
  Subtract3/1 -> [Bit3]
  Divide2/1 -> Floor3/1
  Floor3/1 -> Gain2/1, Divide3/1, Subtract3/1
  Gain2/1 -> Subtract2/2
  Constant9/1 -> Divide/2
  Floor/1 -> Gain/1, Divide1/1, Subtract1/1
  Divide3/1 -> Floor2/1
  Data Type Conversion18/1 -> Bit 0/1
  Divide1/1 -> Floor1/1
  Gain3/1 -> Subtract3/2
  Data Type Conversion13/1 -> Bit 3/1
  Floor1/1 -> Gain1/1, Divide2/1, Subtract2/1
  DecIn/1 -> Data Type Conversion/1
  Floor2/1 -> Gain3/1
  Constant17/1 -> Divide2/2
  [Bit3] -> Data Type Conversion13/1
  Divide/1 -> Floor/1
  [Bit1] -> Data Type Conversion17/1
  Constant18/1 -> Divide3/2
  Subtract/1 -> [Bit0]
  Constant10/1 -> Divide1/2
  [Bit2] -> Data Type Conversion14/1
  Data Type Conversion14/1 -> Bit 2/1
  [Bit0] -> Data Type Conversion18/1
  Subtract2/1 -> [Bit2]
  Gain1/1 -> Subtract1/2
  Subtract1/1 -> [Bit1]
  Gain/1 -> Subtract/2
  Data Type Conversion17/1 -> Bit 1/1

== system SimulinkLibrary/DiscreteSecondOrderSection ==
  u : Inport
  frequency : Inport  Port=2
  Constant : Constant  Value=zeta
  Constant1 : Constant  Value=tau
  Gain1 : Gain  Gain=2
  MATLAB Function : MATLAB Function  Tag=#GainSurfaceTarget_  TreatAsAtomicUnit=on
  Product1 : Product
  Product2 : Product
  Product5 : Product
  Sum : Sum  Inputs=|++
  Sum1 : Sum  Inputs=++|
  Sum2 : Sum  Inputs=+|+
  Sum3 : Sum  Inputs=+|-
  Unit Delay1 : UnitDelay  SampleTime=Ts  HasFrameUpgradeWarning=on
  Unit Delay2 : UnitDelay  SampleTime=Ts  HasFrameUpgradeWarning=on
  y : Outport  VectorParamsAs1DForOutWhenUnconnected=off
  wires:
  Unit Delay1/1 -> Sum/2
  MATLAB Function/3(c) -> Product2/2
  MATLAB Function/2(b) -> Product5/2
  Product2/1 -> Sum3/2
  Constant1/1 -> MATLAB Function/3(tau)
  MATLAB Function/1(a) -> Product1/2
  frequency/1 -> MATLAB Function/1(w)
  Sum1/1 -> Unit Delay1/1
  Sum3/1 -> Unit Delay2/1
  Sum2/1 -> Gain1/1
  Constant/1 -> MATLAB Function/2(zeta)
  Product1/1 -> y/1
  u/1 -> Sum3/1, Sum2/1, Sum/1
  Unit Delay2/1 -> Sum1/2
  Sum/1 -> Product1/1, Product5/1, Product2/1
  Product5/1 -> Sum2/2
  Gain1/1 -> Sum1/1

== system SimulinkLibrary/E2E_1C_CtlCmd ==
  note: DID
      | VehInfo = 0x5B0
      | CtlCmd = 0x60F
      | SftyInfo = 0x8BF
  HvReq : Inport
  IslnMeastDisaCmd : Inport  Port=2
  AliveCounter : Stateflow chart  TreatAsAtomicUnit=on
  CAN Pack : canmsglib/CAN Pack  CANdbFile=C:\Users\mujim\Kleanbus\Engineering - Documents\EV Bus\Components\Battery (Webasto)\batterys Notes\07_VIC_Gen1_0_VEH_CAN.dbc  MsgList=(none)  MsgName=CtlCmd  MsgIDType=Extended (29-bit identifier)  MsgIdentifier=288  MsgLength=8  Remote=off  ApplyMinMax=off  BusOutput=off  SignalInfo={'CtlCmd_Alvctr','8','4','LE','unsigned','Standard','0','1','0','0','255';'CtlCmd_Cks','0','8','LE','unsigned','Standard','0','1','0','0','255';'CtlCmd_DIDNibble','12','4','LE','unsigned','Standard','0','1','0','0','255';'HvReq','16','8','LE','unsigned','Standard','0','1','0','0','255';'IslnMeastDisaCmd','24','2','LE','unsigned','Standard','0','1','0','0','3'}
      settings: SourceProductBaseCode=ME,XP,VN  DataFormat=CANdb specified signals
  CAN Unpack : canmsglib/CAN Unpack  MsgList=(none)  MsgName=CtlCmd  MsgIDType=Extended (29-bit identifier)  MsgIdentifier=288  MsgLength=8  SignalInfo={}  IDPort=off  TimestampPort=off  ErrorPort=off  RemotePort=off  LengthPort=off  StatusPort=off  ApplyMinMax=off
      settings: SourceProductBaseCode=ME,XP,VN  DataFormat=raw data
  CtlCmd_CalcCksm : MATLAB Function  TreatAsAtomicUnit=on
  DID_HiByteLoNibble : Constant  Value=0x6
  DID_LoByte : Constant  Value=0x0F
  Demux : Demux  Outputs=8
  Ground : Ground
  Ground1 : Ground
  Ground2 : Ground
  Terminator{,1..5} (6 alike) : Terminator
  VehInfo_Cks : Outport
  VehInfo_Alvctr : Outport  Port=2
  VehInfo_DIDNibble : Outport  Port=3
  wires:
  [Byte4] -> CtlCmd_CalcCksm/2(VehInfo_Byte4)
  [DID_LoByte] -> CtlCmd_CalcCksm/3(LoByte)
  [Byte3] -> CtlCmd_CalcCksm/1(VehInfo_Byte3)
  Ground1/1 -> CAN Pack/3
  Demux/7 -> Terminator2/1
  Demux/6 -> Terminator5/1
  Demux/4 -> [Byte4]
  Demux/5 -> Terminator4/1
  [DID_HiByteLoNibble] -> CtlCmd_CalcCksm/4(Nibble)
  Demux/3 -> [Byte3]
  CAN Unpack/1 -> Demux/1
  [Alv_Ctr] -> VehInfo_Alvctr/1  "VehInfo_Alvctr"
  CtlCmd_CalcCksm/1(cksm) -> VehInfo_Cks/1  "VehInfo_Cks"
  CAN Pack/1 -> CAN Unpack/1
  Demux/2 -> Terminator1/1
  Demux/8 -> Terminator3/1
  [Alv_Ctr] -> CtlCmd_CalcCksm/5(Alv_Cntr)
  Demux/1 -> Terminator/1
  [IslnMeastDisaCmd] -> CAN Pack/5
  Ground2/1 -> CAN Pack/1
  Ground/1 -> CAN Pack/2
  AliveCounter/1(Alv_Ctr) -> [Alv_Ctr]  "Alv_Ctr"
  DID_HiByteLoNibble/1 -> [DID_HiByteLoNibble]  "DID_HiByteLoNibble"
  IslnMeastDisaCmd/1 -> [IslnMeastDisaCmd]  "IslnMeastDisaCmd"
  [DID_HiByteLoNibble] -> VehInfo_DIDNibble/1  "VehInfo_DIDNibble"
  DID_LoByte/1 -> [DID_LoByte]  "DID_LoByte"
  HvReq/1 -> [HvReq]  "HvReq"
  [HvReq] -> CAN Pack/4

== system SimulinkLibrary/E2E_1C_SftyInfo ==
  note: DID
      | VehInfo = 0x5B0
      | CtlCmd = 0x60F
      | SftyInfo = 0x8BF
  SftyOk : Inport
  CrashDetnNeg : Inport  Port=2
  AliveCounter : Stateflow chart  TreatAsAtomicUnit=on
  CAN Pack : canmsglib/CAN Pack  CANdbFile=C:\Users\mujim\Kleanbus\Engineering - Documents\EV Bus\Components\Battery (Webasto)\batterys Notes\07_VIC_Gen1_0_VEH_CAN.dbc  MsgList=(none)  MsgName=SftyInfo  MsgIDType=Extended (29-bit identifier)  MsgIdentifier=256  MsgLength=8  Remote=off  ApplyMinMax=off  BusOutput=off  SignalInfo={'CrashDetnNeg','18','2','LE','unsigned','Standard','0','1','0','0','3';'SftyInfo_Alvctr','8','4','LE','unsigned','Standard','0','1','0','0','255';'SftyInfo_Cks','0','8','LE','unsigned','Standard','0','1','0','0','255';'SftyInfo_DIDNibble','12','4','LE','unsigned','Standard','0','1','0','0','255';'SftyOk','16','2','LE','unsigned','Standard','0','1','0','0','3'}
      settings: SourceProductBaseCode=ME,XP,VN  DataFormat=CANdb specified signals
  CAN Unpack : canmsglib/CAN Unpack  MsgList=(none)  MsgName=VehInfo  MsgIDType=Extended (29-bit identifier)  MsgIdentifier=256  MsgLength=8  SignalInfo={ 'TAmb', '16', '11', 'LE', 'signed', 'Standard', '0', '0.25', '0', '-256', '255.75'; 'VehInfo_Alvctr', '8', '4', 'LE', 'unsigned', 'Standard', '0', '1', '0', '0', '255'; 'VehInfo_Cks', '0', '8', 'LE', 'unsigned', 'Standard', '0', '1', '0', '0', '255'; 'VehInfo_DIDNibble', '12', '4', 'LE', 'unsigned', 'Standard', '0', '1', '0', '0', '255'; 'VehSpd', '32', '11', 'LE', 'signed', 'Standard', '0', '0.5', '0', '-512', '511.5' }  IDPort=off  TimestampPort=off  ErrorPort=off  RemotePort=off  LengthPort=off  StatusPort=off  ApplyMinMax=off
      settings: SourceProductBaseCode=ME,XP,VN  DataFormat=raw data
  DID_HiByteLoNibble : Constant  Value=0x8
  DID_LoByte : Constant  Value=0xBF
  Demux : Demux  Outputs=8
  Ground : Ground
  Ground1 : Ground
  Ground2 : Ground
  SftyInfo_CalcCksm : MATLAB Function  TreatAsAtomicUnit=on
  SftyInfo_CalcCksm1 : MATLAB Function  Commented=on  TreatAsAtomicUnit=on
  Terminator{,1..6} (7 alike) : Terminator
  Cksm : Outport
  Alv_Cntr : Outport  Port=2
  DID_Nibble : Outport  Port=3
  wires:
  AliveCounter/1(Alv_Ctr) -> [Alv_Ctr]  "Alv_Ctr"
  [Alv_Ctr] -> Alv_Cntr/1  "Alv_Ctr"
  DID_LoByte/1 -> [DID_LoByte]  "DID_LoByte"
  DID_HiByteLoNibble/1 -> [DID_HiByteLoNibble]  "DID_HiByteLoNibble"
  [DID_HiByteLoNibble] -> DID_Nibble/1  "DID_Nibble"
  SftyOk/1 -> [SftyOk]  "SftyOk"
  CrashDetnNeg/1 -> [CrashDetnNeg]  "CrashDetnNeg"
  [DID_HiByteLoNibble] -> SftyInfo_CalcCksm/3(Nibble)
  [DID_LoByte] -> SftyInfo_CalcCksm/2(LoByte)
  [Alv_Ctr] -> SftyInfo_CalcCksm/4(Alv_Cntr)
  SftyInfo_CalcCksm/1(cksm) -> Cksm/1  "Cksm"
  CAN Pack/1 -> CAN Unpack/1
  [SftyOk] -> CAN Pack/5
  [CrashDetnNeg] -> CAN Pack/1
  Ground/1 -> CAN Pack/2
  Ground1/1 -> CAN Pack/3
  Ground2/1 -> CAN Pack/4
  CAN Unpack/1 -> Demux/1
  Demux/1 -> Terminator/1
  Demux/2 -> Terminator1/1
  Demux/3 -> SftyInfo_CalcCksm/1(SftyInfo_byte3)
  Demux/5 -> Terminator3/1
  Demux/4 -> Terminator2/1
  Demux/7 -> Terminator4/1
  Demux/8 -> Terminator5/1
  Demux/6 -> Terminator6/1

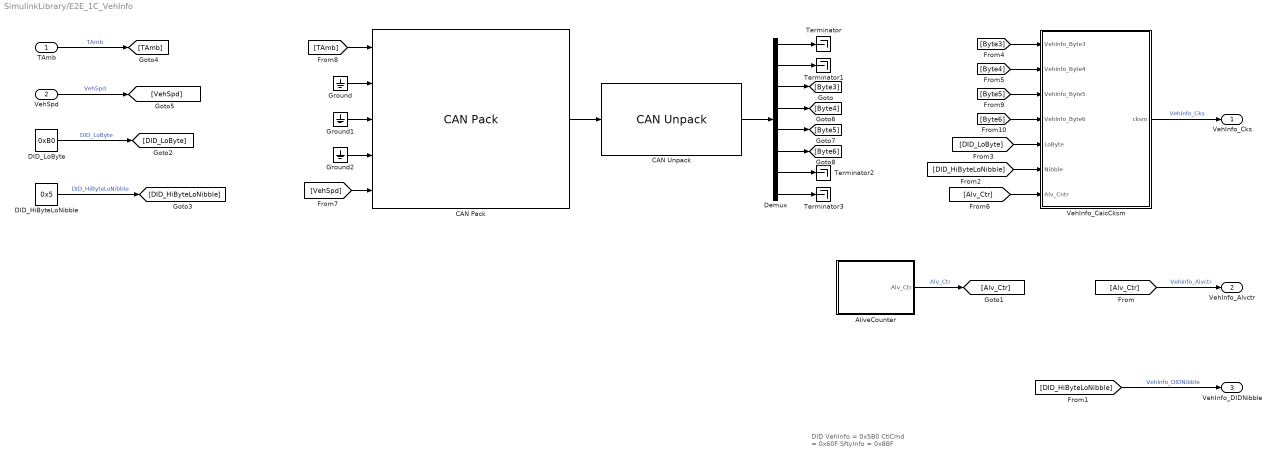
== system SimulinkLibrary/E2E_1C_VehInfo ==
  note: DID
      | VehInfo = 0x5B0
      | CtlCmd = 0x60F
      | SftyInfo = 0x8BF
  TAmb : Inport
  VehSpd : Inport  Port=2
  AliveCounter : Stateflow chart  TreatAsAtomicUnit=on
  CAN Pack : canmsglib/CAN Pack  CANdbFile=C:\Users\mujim\Kleanbus\Engineering - Documents\EV Bus\Components\Battery (Webasto)\batterys Notes\07_VIC_Gen1_0_VEH_CAN.dbc  MsgList=(none)  MsgName=VehInfo  MsgIDType=Extended (29-bit identifier)  MsgIdentifier=257  MsgLength=8  Remote=off  ApplyMinMax=off  BusOutput=off  SignalInfo={'TAmb','16','11','LE','signed','Standard','0','0.25','0','-256','255.75';'VehInfo_Alvctr','8','4','LE','unsigned','Standard','0','1','0','0','255';'VehInfo_Cks','0','8','LE','unsigned','Standard','0','1','0','0','255';'VehInfo_DIDNibble','12','4','LE','unsigned','Standard','0','1','0','0','255';'VehSpd','32','11','LE','signed','Standard','0','0.5','0','-512','511.5'}
      settings: SourceProductBaseCode=ME,XP,VN  DataFormat=CANdb specified signals
  CAN Unpack : canmsglib/CAN Unpack  MsgList=(none)  MsgName=VehInfo  MsgIDType=Extended (29-bit identifier)  MsgIdentifier=257  MsgLength=8  SignalInfo={}  IDPort=off  TimestampPort=off  ErrorPort=off  RemotePort=off  LengthPort=off  StatusPort=off  ApplyMinMax=off
      settings: SourceProductBaseCode=ME,XP,VN  DataFormat=raw data
  DID_HiByteLoNibble : Constant  Value=0x5
  DID_LoByte : Constant  Value=0xB0
  Demux : Demux  Outputs=8
  Ground : Ground
  Ground1 : Ground
  Ground2 : Ground
  Terminator{,1..3} (4 alike) : Terminator
  VehInfo_CalcCksm : MATLAB Function  TreatAsAtomicUnit=on
  VehInfo_Cks : Outport
  VehInfo_Alvctr : Outport  Port=2
  VehInfo_DIDNibble : Outport  Port=3
  wires:
  VehInfo_CalcCksm/1(cksm) -> VehInfo_Cks/1  "VehInfo_Cks"
  TAmb/1 -> [TAmb]  "TAmb"
  [Alv_Ctr] -> VehInfo_CalcCksm/7(Alv_Cntr)
  [DID_HiByteLoNibble] -> VehInfo_DIDNibble/1  "VehInfo_DIDNibble"
  DID_LoByte/1 -> [DID_LoByte]  "DID_LoByte"
  VehSpd/1 -> [VehSpd]  "VehSpd"
  [DID_LoByte] -> VehInfo_CalcCksm/5(LoByte)
  [Alv_Ctr] -> VehInfo_Alvctr/1  "VehInfo_Alvctr"
  [DID_HiByteLoNibble] -> VehInfo_CalcCksm/6(Nibble)
  AliveCounter/1(Alv_Ctr) -> [Alv_Ctr]  "Alv_Ctr"
  DID_HiByteLoNibble/1 -> [DID_HiByteLoNibble]  "DID_HiByteLoNibble"
  [VehSpd] -> CAN Pack/5
  [TAmb] -> CAN Pack/1
  Ground/1 -> CAN Pack/2
  Ground1/1 -> CAN Pack/3
  Ground2/1 -> CAN Pack/4
  CAN Pack/1 -> CAN Unpack/1
  CAN Unpack/1 -> Demux/1
  Demux/3 -> [Byte3]
  [Byte3] -> VehInfo_CalcCksm/1(VehInfo_Byte3)
  Demux/4 -> [Byte4]
  [Byte4] -> VehInfo_CalcCksm/2(VehInfo_Byte4)
  Demux/5 -> [Byte5]
  Demux/6 -> [Byte6]
  [Byte5] -> VehInfo_CalcCksm/3(VehInfo_Byte5)
  [Byte6] -> VehInfo_CalcCksm/4(VehInfo_Byte6)
  Demux/1 -> Terminator/1
  Demux/2 -> Terminator1/1
  Demux/8 -> Terminator3/1
  Demux/7 -> Terminator2/1

== system SimulinkLibrary/J193922ByteParser ==
  Data_In : Inport
  Demux : Demux  Outputs=22
  Terminator{1..2,6,11..19,33..34} (14 alike) : Terminator
  Byte0 : Outport
  Byte1 : Outport  Port=2
  Byte2 : Outport  Port=3
  Byte3 : Outport  Port=4
  Byte4 : Outport  Port=5
  Byte5 : Outport  Port=6
  Byte6 : Outport  Port=7
  Byte7 : Outport  Port=8
  wires:
  Demux/4 -> Byte3/1
  Demux/1 -> Byte0/1
  Demux/3 -> Byte2/1
  Demux/6 -> Byte5/1
  Demux/8 -> Byte7/1
  Demux/7 -> Byte6/1
  Demux/2 -> Byte1/1
  Demux/5 -> Byte4/1
  Data_In/1 -> Demux/1
  Demux/9 -> Terminator2/1
  Demux/12 -> Terminator1/1
  Demux/10 -> Terminator6/1
  Demux/11 -> Terminator11/1
  Demux/16 -> Terminator13/1
  Demux/17 -> Terminator15/1
  Demux/13 -> Terminator17/1
  Demux/18 -> Terminator16/1
  Demux/19 -> Terminator14/1
  Demux/14 -> Terminator18/1
  Demux/15 -> Terminator19/1
  Demux/20 -> Terminator12/1
  Demux/21 -> Terminator33/1
  Demux/22 -> Terminator34/1

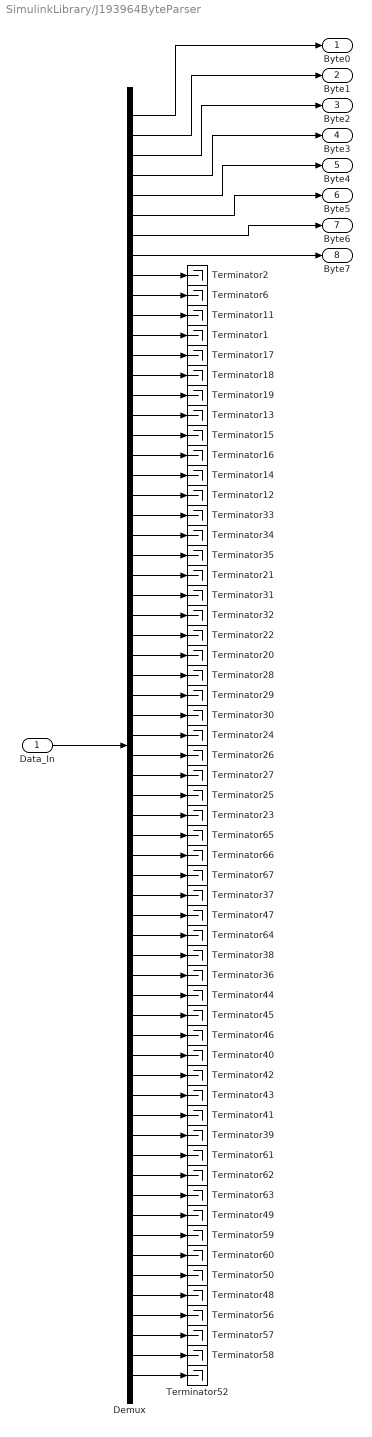
== system SimulinkLibrary/J193964ByteParser ==
  Data_In : Inport
  Demux : Demux  Outputs=64
  Terminator{1..2,6,11..50,52,56..67} (56 alike) : Terminator
  Byte0 : Outport
  Byte1 : Outport  Port=2
  Byte2 : Outport  Port=3
  Byte3 : Outport  Port=4
  Byte4 : Outport  Port=5
  Byte5 : Outport  Port=6
  Byte6 : Outport  Port=7
  Byte7 : Outport  Port=8
  wires:
  Demux/4 -> Byte3/1
  Demux/1 -> Byte0/1
  Demux/3 -> Byte2/1
  Demux/6 -> Byte5/1
  Demux/8 -> Byte7/1
  Demux/7 -> Byte6/1
  Demux/2 -> Byte1/1
  Demux/5 -> Byte4/1
  Data_In/1 -> Demux/1
  Demux/9 -> Terminator2/1
  Demux/12 -> Terminator1/1
  Demux/10 -> Terminator6/1
  Demux/11 -> Terminator11/1
  Demux/16 -> Terminator13/1
  Demux/17 -> Terminator15/1
  Demux/13 -> Terminator17/1
  Demux/18 -> Terminator16/1
  Demux/19 -> Terminator14/1
  Demux/14 -> Terminator18/1
  Demux/15 -> Terminator19/1
  Demux/20 -> Terminator12/1
  Demux/34 -> Terminator27/1
  Demux/21 -> Terminator33/1
  Demux/33 -> Terminator26/1
  Demux/24 -> Terminator21/1
  Demux/22 -> Terminator34/1
  Demux/23 -> Terminator35/1
  Demux/25 -> Terminator31/1
  Demux/26 -> Terminator32/1
  Demux/27 -> Terminator22/1
  Demux/32 -> Terminator24/1
  Demux/29 -> Terminator28/1
  Demux/31 -> Terminator30/1
  Demux/35 -> Terminator25/1
  Demux/36 -> Terminator23/1
  Demux/30 -> Terminator29/1
  Demux/28 -> Terminator20/1
  Demux/50 -> Terminator43/1
  Demux/37 -> Terminator65/1
  Demux/49 -> Terminator42/1
  Demux/40 -> Terminator37/1
  Demux/38 -> Terminator66/1
  Demux/39 -> Terminator67/1
  Demux/42 -> Terminator64/1
  Demux/43 -> Terminator38/1
  Demux/45 -> Terminator44/1
  Demux/48 -> Terminator40/1
  Demux/47 -> Terminator46/1
  Demux/51 -> Terminator41/1
  Demux/46 -> Terminator45/1
  Demux/52 -> Terminator39/1
  Demux/53 -> Terminator61/1
  Demux/56 -> Terminator49/1
  Demux/60 -> Terminator48/1
  Demux/64 -> Terminator52/1
  Demux/59 -> Terminator50/1
  Demux/61 -> Terminator56/1
  Demux/54 -> Terminator62/1
  Demux/58 -> Terminator60/1
  Demux/57 -> Terminator59/1
  Demux/55 -> Terminator63/1
  Demux/41 -> Terminator47/1
  Demux/62 -> Terminator57/1
  Demux/63 -> Terminator58/1
  Demux/44 -> Terminator36/1

== system SimulinkLibrary/LatchSetDom ==
  Set : Inport
  Reset : Inport  Port=2
  Signal in : Inport  Port=3
  Signal out : Outport

== system SimulinkLibrary/MinMaxSat ==
  up : Inport
  u : Inport  Port=2
  lo : Inport  Port=3
  LowerRelop1 : RelationalOperator  DisableCoverage=on  Operator=>  OutDataTypeStr=boolean  RndMeth=Nearest
  Switch : Switch  Criteria=u2 ~= 0  OutDataTypeStr=Inherit: Inherit via back propagation  ZeroCross=off
  Switch1 : Switch  Criteria=u2 ~= 0
  UpperRelop : RelationalOperator  DisableCoverage=on  Operator=<  OutDataTypeStr=boolean  RndMeth=Nearest
  y : Outport
  wires:
  Switch/1 -> Switch1/3
  LowerRelop1/1 -> Switch1/2
  UpperRelop/1 -> Switch/2
  Switch1/1 -> y/1
  u/1 -> LowerRelop1/1, Switch/3, UpperRelop/1
  up/1 -> Switch1/1, LowerRelop1/2
  lo/1 -> Switch/1, UpperRelop/2

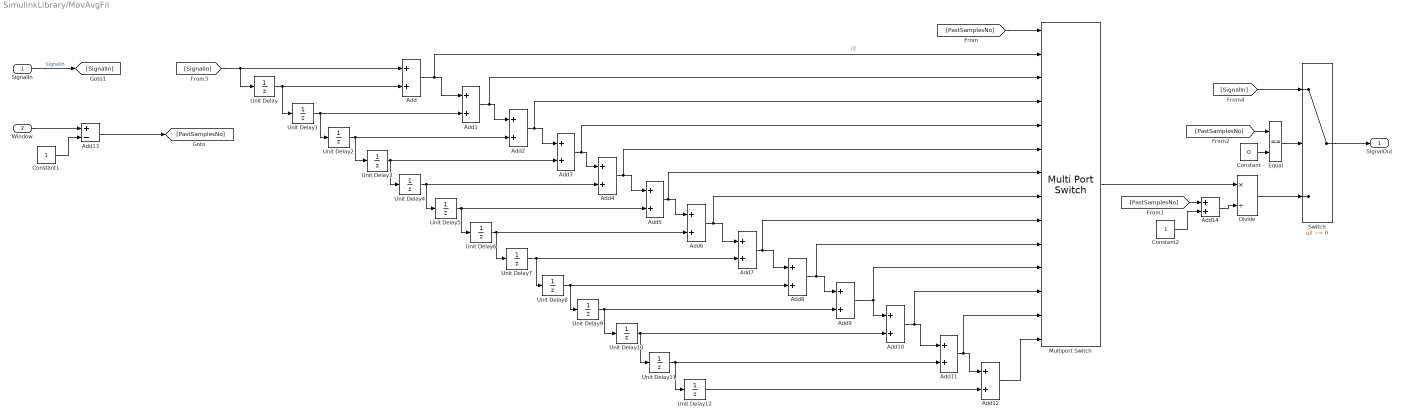
== system SimulinkLibrary/MovAvgFil ==
  note: /2
  SignalIn : Inport
  Window : Inport  Port=2
  Add{,1..12,14} (14 alike) : Sum
  Add13 : Sum  Inputs=+-
  Constant : Constant  Value=0
  Constant1 : Constant
  Constant2 : Constant
  Divide : Product  Inputs=*/
  Equal : RelationalOperator  Operator===  OutDataTypeStr=boolean  RndMeth=Simplest
  Multiport Switch : MultiPortSwitch  Inputs=13
  Switch : Switch  Criteria=u2 ~= 0  RndMeth=Zero
  Unit Delay{,1..12} (13 alike) : UnitDelay  SampleTime=-1  HasFrameUpgradeWarning=on
  SIgnalOut : Outport
  wires:
  Divide/1 -> Switch/3
  [SignalIn] -> Switch/1
  Switch/1 -> SIgnalOut/1
  Equal/1 -> Switch/2
  [SignalIn] -> Unit Delay/1, Add/1
  Constant/1 -> Equal/2
  [PastSamplesNo] -> Equal/1
  [PastSamplesNo] -> Multiport Switch/1
  Multiport Switch/1 -> Divide/1
  Add12/1 -> Multiport Switch/14
  Add11/1 -> Multiport Switch/13, Add12/1
  Add10/1 -> Multiport Switch/12, Add11/1
  Unit Delay11/1 -> Unit Delay12/1, Add11/2
  Add9/1 -> Add10/1, Multiport Switch/11
  Add8/1 -> Multiport Switch/10, Add9/1
  Add7/1 -> Multiport Switch/9, Add8/1
  Add6/1 -> Multiport Switch/8, Add7/1
  Add5/1 -> Multiport Switch/7, Add6/1
  Add4/1 -> Multiport Switch/6, Add5/1
  Add3/1 -> Multiport Switch/5, Add4/1
  Add2/1 -> Multiport Switch/4, Add3/1
  Add1/1 -> Multiport Switch/3, Add2/1
  Add/1 -> Multiport Switch/2, Add1/1
  Unit Delay4/1 -> Unit Delay5/1, Add4/2
  Unit Delay2/1 -> Unit Delay3/1, Add2/2
  Unit Delay7/1 -> Add7/2, Unit Delay8/1
  Unit Delay8/1 -> Unit Delay9/1, Add8/2
  Unit Delay3/1 -> Unit Delay4/1, Add3/2
  Unit Delay12/1 -> Add12/2
  Unit Delay6/1 -> Add6/2, Unit Delay7/1
  SignalIn/1 -> [SignalIn]  "SignalIn"
  Unit Delay10/1 -> Unit Delay11/1, Add10/2
  Unit Delay1/1 -> Unit Delay2/1, Add1/2
  Unit Delay/1 -> Unit Delay1/1, Add/2
  Unit Delay9/1 -> Unit Delay10/1, Add9/2
  Unit Delay5/1 -> Add5/2, Unit Delay6/1
  Add13/1 -> [PastSamplesNo]
  Window/1 -> Add13/1
  Constant1/1 -> Add13/2
  Constant2/1 -> Add14/2
  [PastSamplesNo] -> Add14/1
  Add14/1 -> Divide/2

== system SimulinkLibrary/RangeCheck ==
  In : Inport
  UpLim : Inport  Port=2
  LowLim : Inport  Port=3
  AND : Logic  AllPortsSameDT=off  OutDataTypeStr=boolean
  Lower Test : RelationalOperator  DisableCoverage=on  OutDataTypeStr=boolean  ZeroCross=off  RndMeth=Nearest
  Upper Test : RelationalOperator  DisableCoverage=on  Operator=<=  OutDataTypeStr=boolean  ZeroCross=off  RndMeth=Nearest
  Out : Outport
  wires:
  UpLim/1 -> Upper Test/2  "UpLim"
  Lower Test/1 -> AND/2
  AND/1 -> Out/1  "Out"
  LowLim/1 -> Lower Test/2  "LowLim"
  Upper Test/1 -> AND/1
  In/1 -> [In]
  [In] -> Lower Test/1
  [In] -> Upper Test/1
